simulink model "CruiseControl"  (R2020a)
settings: Solver=VariableStepAuto  StartTime=0.0  StopTime=10.0  RelTol=1e-3
undefined symbols (not defined in the file): b, m
settings Model: Creator=Admin  LastModifiedBy=Admin

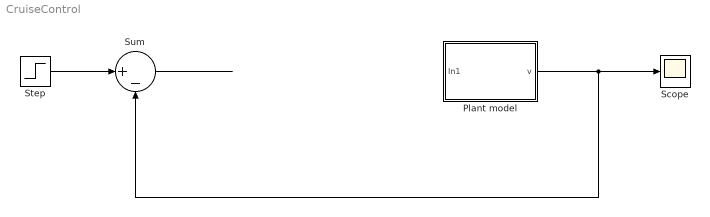
== system CruiseControl ==
  Plant model : Subsystem
  Scope : Scope
  Step : Step  SampleTime=0
  Sum : Sum  Inputs=|+-
  wires:
  ? -> Plant model/1(In1)
  Plant model/1(v) -> Sum/2, Scope/1
  Step/1 -> Sum/1
  Sum/1 -> ?

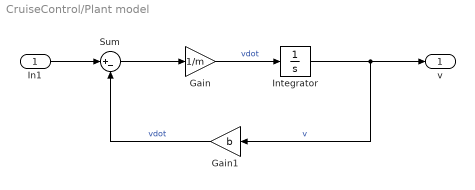
== system CruiseControl/Plant model ==
  In1 : Inport
  Gain : Gain  Gain=1/m
  Gain1 : Gain  Gain=b
  Integrator : Integrator
  Sum : Sum  Inputs=|+-
  v : Outport
  wires:
  Gain/1 -> Integrator/1  "vdot"
  Integrator/1 -> v/1, Gain1/1  "v"
  Sum/1 -> Gain/1
  In1/1 -> Sum/1
  Gain1/1 -> Sum/2  "vdot"
